simulink model "zerocross"  (Simulink 10.0)
settings: Solver=ode45  StartTime=0.0  StopTime=10.0  RelTol=1e-3  EnableMultiTasking=on
settings Model: Creator=bhisma  LastModifiedBy=bhisma
settings DataIOCC: SignalLoggingSaveFormat=ModelDataLogs
settings OptimizationCC: BlockReduction=off  BooleanDataType=off  DefaultParameterBehavior=Inlined  LifeSpan=auto
settings DebuggingCC: SaveWithParameterizedLinksMsg=none  SignalResolutionControl=TryResolveAllWithWarning  MultiTaskDSMMsg=warning  MultiTaskCondExecSysMsg=none  SFUnexpectedBacktrackingDiag=error  SFNoUnconditionalDefaultTransitionDiag=error  SFExecutionAtInitializationDiag=warning  ArithmeticOperatorsInVariantConditions=error
settings HardwareCC: ProdBitPerPointer=64  ProdBitPerSizeT=64  ProdBitPerPtrDiffT=64  ProdLargestAtomicFloat=Float  ProdIntDivRoundTo=Zero  ProdEndianess=LittleEndian  ProdWordSize=64  ProdHWDeviceType=Intel->x86-64 (Windows64)  TargetUnknown=on
settings SFSimCC: SimUseLocalCustomCode=on  CustomCodeUndefinedFunction=FilterOut
settings RTWCC: RTWUseLocalCustomCode=on
settings CodeAppCC: StateflowObjectComments=off
settings GRTTargetCC: TargetLangStandard=C99 (ISO)
settings ConfigComp: CovMetricSettings=dwe  CovSaveCumulativeToWorkspaceVar=off  CovSaveSingleToWorkspaceVar=off

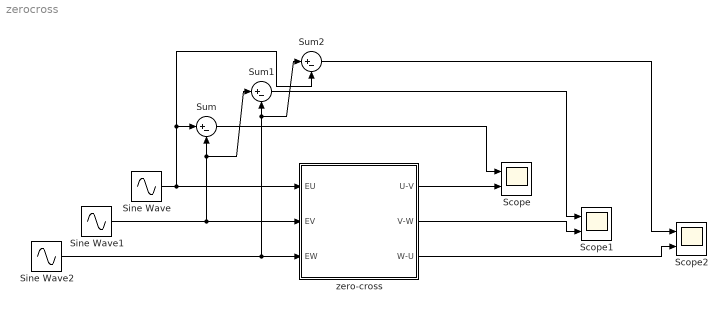
== system zerocross ==
  Scope : Scope  NumInputPorts=2
  Scope1 : Scope  NumInputPorts=2
  Scope2 : Scope  NumInputPorts=2
  Sine Wave : Sin  Frequency=10  SampleTime=0
  Sine Wave1 : Sin  Frequency=10  Phase=2*pi/3  SampleTime=0
  Sine Wave2 : Sin  Frequency=10  Phase=-2*pi/3  SampleTime=0
  Sum : Sum  Inputs=|+-  SaturateOnIntegerOverflow=on  InputSameDT=on  OutDataTypeStr=Inherit: Same as first input
  Sum1 : Sum  Inputs=|+-  SaturateOnIntegerOverflow=on  InputSameDT=on  OutDataTypeStr=Inherit: Same as first input
  Sum2 : Sum  Inputs=|+-  SaturateOnIntegerOverflow=on  InputSameDT=on  OutDataTypeStr=Inherit: Same as first input
  zero-cross : Subsystem
      mask help: The block detects the zero crossing of the inputs. For accurate results use the rising edge only.
  wires:
  Sine Wave/1 -> zero-cross/1(EU), Sum/1, Sum2/2
  Sine Wave1/1 -> zero-cross/2(EV), Sum/2, Sum1/1
  Sine Wave2/1 -> zero-cross/3(EW), Sum1/2, Sum2/1
  zero-cross/1(U-V) -> Scope/2
  Sum/1 -> Scope/1
  Sum1/1 -> Scope1/1
  zero-cross/2(V-W) -> Scope1/2
  Sum2/1 -> Scope2/1
  zero-cross/3(W-U) -> Scope2/2

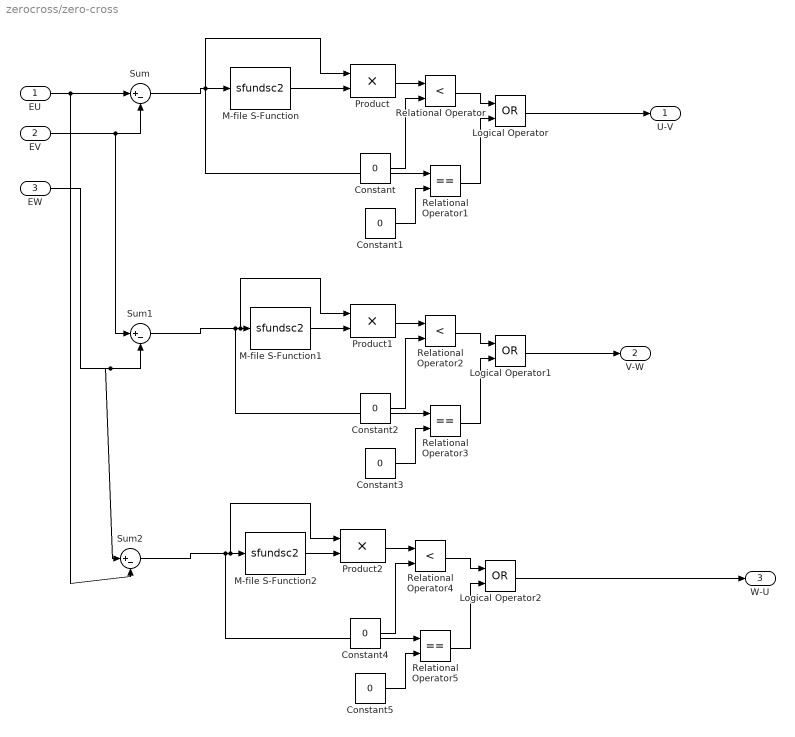
== system zerocross/zero-cross ==
  EU : Inport
  EV : Inport  Port=2
  EW : Inport  Port=3
  Constant{,1..5} (6 alike) : Constant  Value=0
  Logical Operator : Logic  Operator=OR
  Logical Operator1 : Logic  Operator=OR
  Logical Operator2 : Logic  Operator=OR
  M-file S-Function : S-Function  FunctionName=sfundsc2  SFunctionDeploymentMode=off  EnableBusSupport=off  mask(S-function: sfun_dsc2){}
      mask help: This is a M-file S-function which demonstrates how toimplement an unit delay.
      mask Display: disp('Unit delay')
  M-file S-Function1 : S-Function  FunctionName=sfundsc2  SFunctionDeploymentMode=off  EnableBusSupport=off  mask(S-function: sfun_dsc2){}
      mask help: This is a M-file S-function which demonstrates how toimplement an unit delay.
      mask Display: disp('Unit delay')
  M-file S-Function2 : S-Function  FunctionName=sfundsc2  SFunctionDeploymentMode=off  EnableBusSupport=off  mask(S-function: sfun_dsc2){}
      mask help: This is a M-file S-function which demonstrates how toimplement an unit delay.
      mask Display: disp('Unit delay')
  Product : Product  SaturateOnIntegerOverflow=on  RndMeth=Zero  InputSameDT=on  OutDataTypeStr=Inherit: Same as first input
  Product1 : Product  SaturateOnIntegerOverflow=on  RndMeth=Zero  InputSameDT=on  OutDataTypeStr=Inherit: Same as first input
  Product2 : Product  SaturateOnIntegerOverflow=on  RndMeth=Zero  InputSameDT=on  OutDataTypeStr=Inherit: Same as first input
  Relational Operator : RelationalOperator  Operator=<  RndMeth=Nearest  InputSameDT=on
  Relational Operator1 : RelationalOperator  Operator===  RndMeth=Nearest  InputSameDT=on
  Relational Operator2 : RelationalOperator  Operator=<  RndMeth=Nearest  InputSameDT=on
  Relational Operator3 : RelationalOperator  Operator===  RndMeth=Nearest  InputSameDT=on
  Relational Operator4 : RelationalOperator  Operator=<  RndMeth=Nearest  InputSameDT=on
  Relational Operator5 : RelationalOperator  Operator===  RndMeth=Nearest  InputSameDT=on
  Sum : Sum  Inputs=|+-  SaturateOnIntegerOverflow=on  InputSameDT=on  OutDataTypeStr=Inherit: Same as first input
  Sum1 : Sum  Inputs=|+-  SaturateOnIntegerOverflow=on  InputSameDT=on  OutDataTypeStr=Inherit: Same as first input
  Sum2 : Sum  Inputs=|+-  SaturateOnIntegerOverflow=on  InputSameDT=on  OutDataTypeStr=Inherit: Same as first input
  U-V : Outport
  V-W : Outport  Port=2
  W-U : Outport  Port=3
  wires:
  Sum/1 -> Relational Operator1/1, Product/1, M-file S-Function/1
  M-file S-Function/1 -> Product/2
  Product/1 -> Relational Operator/1
  Constant/1 -> Relational Operator/2
  Constant1/1 -> Relational Operator1/2
  Relational Operator/1 -> Logical Operator/1
  Relational Operator1/1 -> Logical Operator/2
  Logical Operator/1 -> U-V/1
  EU/1 -> Sum/1, Sum2/2
  EV/1 -> Sum/2, Sum1/1
  Sum1/1 -> Relational Operator3/1, Product1/1, M-file S-Function1/1
  M-file S-Function1/1 -> Product1/2
  Product1/1 -> Relational Operator2/1
  Constant2/1 -> Relational Operator2/2
  Constant3/1 -> Relational Operator3/2
  Relational Operator2/1 -> Logical Operator1/1
  Relational Operator3/1 -> Logical Operator1/2
  Logical Operator1/1 -> V-W/1
  EW/1 -> Sum1/2, Sum2/1
  Sum2/1 -> M-file S-Function2/1, Product2/1, Relational Operator5/1
  M-file S-Function2/1 -> Product2/2
  Product2/1 -> Relational Operator4/1
  Constant4/1 -> Relational Operator4/2
  Constant5/1 -> Relational Operator5/2
  Relational Operator4/1 -> Logical Operator2/1
  Relational Operator5/1 -> Logical Operator2/2
  Logical Operator2/1 -> W-U/1
